simulink model "parallel_controller_mar_10"  (R2017b)
settings: Solver=FixedStepAuto  StartTime=0.0  StopTime=10  FixedStep=0.0001  RelTol=1e-3
InitFcn:
  | ra = 4;
  | jm = 0.0000218;
  | rm = 0.7/100;
  | dsm = 62.892;
  | kt = 0.138;
  | ke = kt;
  | ms = 0.93;
  | hl = 1.5 / 100;
  | Lr = 24.1 / 100;
  | Lcm = hl / 2 + Lr;
  | ml =0.182;
  | mr = 0.085;
  | rl = 20.125 / 1000;
  | Jp =1/3 * mr * Lr^2 + 1/2*ml*rl^2 + ml * Lcm ^ 2;
  | Dp = 0.007;
  | g = 9.82;
StartFcn:
  | ra = 4;
  | jm = 0.0000218;
  | rm = 0.7/100;
  | dsm = 62.892;
  | kt = 0.138;
  | ke = kt;
  | ms = 0.93;
undefined symbols (not defined in the file): direction_sign, distance, Ka, Kd, Ki, Kp, National_Instruments, PCI, saturation_lower, saturation_upper, tau, theta_max
libraries: sldrtlib x4
settings Model: Creator=labadmin  LastModifiedBy=labadmin
settings RTWCC: SystemTargetFile=sldrt.tlc  TemplateMakefile=sldrt.tmf  Description=Simulink Desktop Real-Time  RTWCompilerOptimization=on
settings CodeAppCC: MaxIdLength=95
settings SimulinkDesktopRealTimeCC: TargetPreCompLibLocation=C:\Program Files\MATLAB\R2017b\toolbox\sldrt\lib\win64

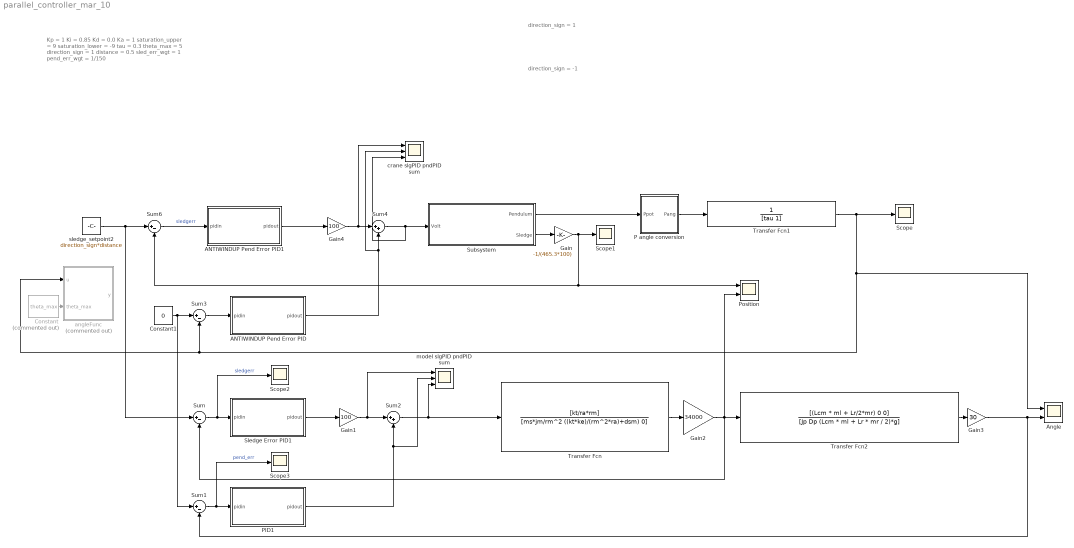
== system parallel_controller_mar_10 ==
  note: Kp = 1
      | Ki = 0.85
      | Kd = 0.0
      | Ka = 1
      | saturation_upper = 9
      | saturation_lower = -9
      | tau = 0.3
      | theta_max = 5
      | direction_sign = 1
      | distance = 0.5
      | sled_err_wgt = 1
      | pend_err_wgt = 1/150
  note: direction_sign = -1
  note: direction_sign = 1
  ANTIWINDUP Pend Error PID : Subsystem
  ANTIWINDUP Pend Error PID1 : Subsystem
  Angle : Scope  NumInputPorts=2
  Constant : Constant  Commented=on  Value=theta_max
  Constant1 : Constant  Value=0
  Gain : Gain  Gain=-1/(465.3*100)
  Gain1 : Gain  Gain=100
  Gain2 : Gain  Gain=34000
  Gain3 : Gain  Gain=30
  Gain4 : Gain  Gain=100
  P angle conversion : Subsystem
  PID1 : Subsystem
  Position : Scope  NumInputPorts=2
  Scope{,1..3} (4 alike) : Scope
  Sledge Error PID1 : Subsystem
  Subsystem : Subsystem
  Sum{,1,3,6} (4 alike) : Sum  Inputs=|+-
  Sum2 : Sum  Inputs=|++
  Sum4 : Sum  Inputs=|++
  Transfer Fcn : TransferFcn  Numerator=[kt/ra*rm]  Denominator=[ms*jm/rm^2 ((kt*ke)/(rm^2*ra)+dsm) 0]
  Transfer Fcn1 : TransferFcn  Denominator=[tau 1]
  Transfer Fcn2 : TransferFcn  Numerator=[(Lcm * ml + Lr/2*mr) 0 0]  Denominator=[Jp Dp (Lcm * ml + Lr * mr / 2)*g]
  "angleFunc " : MATLAB Function  Commented=on  TreatAsAtomicUnit=on
  crane slgPID pndPID sum : Scope  NumInputPorts=3
  model slgPID pndPID sum : Scope  NumInputPorts=3
  sledge_setpoint2 : Constant  Value=direction_sign*distance
  wires:
  Gain/1 -> Sum6/2, Position/1, Scope1/1
  Subsystem/1(Pendulum) -> P angle conversion/1(Ppot)
  Subsystem/2(Sledge) -> Gain/1
  Transfer Fcn/1 -> Gain2/1
  Gain2/1 -> Sum/2, Position/2, Transfer Fcn2/1
  Gain3/1 -> Sum1/2, Angle/2
  sledge_setpoint2/1 -> Sum/1, Sum6/1
  PID1/1(pidout) -> model slgPID pndPID sum/2, Sum2/2
  Sum6/1 -> ANTIWINDUP Pend Error PID1/1(pidin)  "sledgerr"
  P angle conversion/1(Pang) -> Transfer Fcn1/1
  Sum2/1 -> model slgPID pndPID sum/3, Transfer Fcn/1
  Transfer Fcn1/1 -> Scope/1, Angle/1, "angleFunc "/1(u), Sum3/2
  Constant/1 -> "angleFunc "/2(theta_max)
  Constant1/1 -> Sum1/1, Sum3/1
  Transfer Fcn2/1 -> Gain3/1
  Sum3/1 -> ANTIWINDUP Pend Error PID/1(pidin)
  ANTIWINDUP Pend Error PID1/1(pidout) -> Gain4/1
  ANTIWINDUP Pend Error PID/1(pidout) -> crane slgPID pndPID sum/2, Sum4/2
  Sum/1 -> Scope2/1, Sledge Error PID1/1(pidin)  "sledgerr"
  Sledge Error PID1/1(pidout) -> Gain1/1
  Sum1/1 -> Scope3/1, PID1/1(pidin)  "pend_err"
  Gain1/1 -> model slgPID pndPID sum/1, Sum2/1
  Sum4/1 -> crane slgPID pndPID sum/3, Subsystem/1(Volt)
  Gain4/1 -> crane slgPID pndPID sum/1, Sum4/1

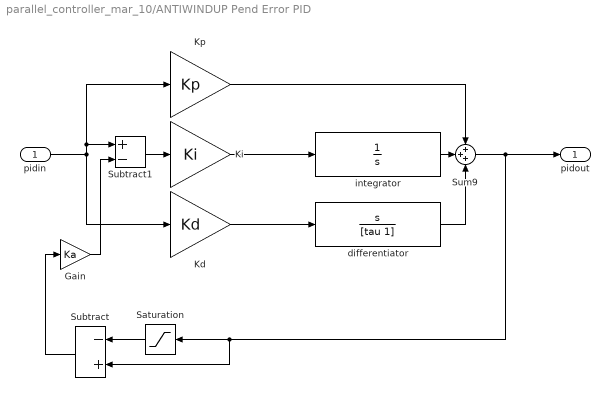
== system parallel_controller_mar_10/ANTIWINDUP Pend Error PID ==
  pidin : Inport
  Gain : Gain  Gain=Ka
  Kd : Gain  Gain=Kd
  Ki : Gain  Gain=Ki
  Kp : Gain  Gain=Kp
  Saturation : Saturate  UpperLimit=saturation_upper  LowerLimit=saturation_lower
  Subtract : Sum  Inputs=-+
  Subtract1 : Sum  Inputs=+-
  Sum9 : Sum  Inputs=+++
  differentiator : TransferFcn  Numerator=[1 0]  Denominator=[tau 1]
  integrator : TransferFcn  Denominator=[1 0]
  pidout : Outport
  wires:
  pidin/1 -> Kp/1, Subtract1/1, Kd/1
  Sum9/1 -> Subtract/2, Saturation/1, pidout/1
  Kd/1 -> differentiator/1
  Ki/1 -> integrator/1
  Kp/1 -> Sum9/1
  integrator/1 -> Sum9/2
  differentiator/1 -> Sum9/3
  Saturation/1 -> Subtract/1
  Subtract/1 -> Gain/1
  Gain/1 -> Subtract1/2
  Subtract1/1 -> Ki/1

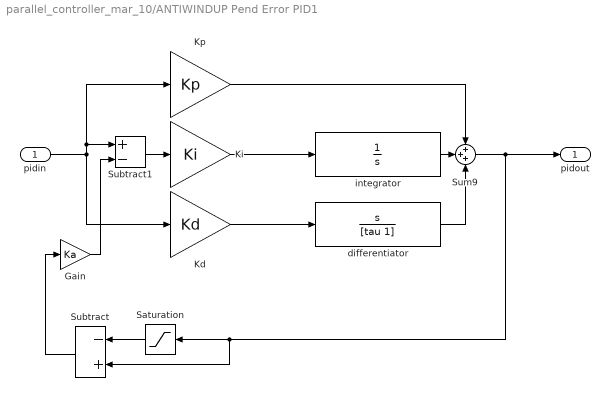
== system parallel_controller_mar_10/ANTIWINDUP Pend Error PID1 ==
  pidin : Inport
  Gain : Gain  Gain=Ka
  Kd : Gain  Gain=Kd
  Ki : Gain  Gain=Ki
  Kp : Gain  Gain=Kp
  Saturation : Saturate  UpperLimit=saturation_upper  LowerLimit=saturation_lower
  Subtract : Sum  Inputs=-+
  Subtract1 : Sum  Inputs=+-
  Sum9 : Sum  Inputs=+++
  differentiator : TransferFcn  Numerator=[1 0]  Denominator=[tau 1]
  integrator : TransferFcn  Denominator=[1 0]
  pidout : Outport
  wires:
  pidin/1 -> Kp/1, Subtract1/1, Kd/1
  Sum9/1 -> Subtract/2, Saturation/1, pidout/1
  Kd/1 -> differentiator/1
  Ki/1 -> integrator/1
  Kp/1 -> Sum9/1
  integrator/1 -> Sum9/2
  differentiator/1 -> Sum9/3
  Saturation/1 -> Subtract/1
  Subtract/1 -> Gain/1
  Gain/1 -> Subtract1/2
  Subtract1/1 -> Ki/1

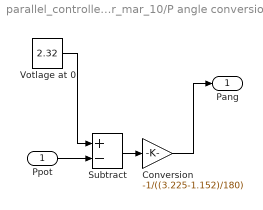
== system parallel_controller_mar_10/P angle conversion ==
  Ppot : Inport
  Conversion : Gain  Gain=-1/((3.225-1.152)/180)
  Subtract : Sum  Inputs=+-
  "Votlage at 0 " : Constant  Value=2.32
  Pang : Outport
  wires:
  Subtract/1 -> Conversion/1
  Ppot/1 -> Subtract/2
  "Votlage at 0 "/1 -> Subtract/1
  Conversion/1 -> Pang/1

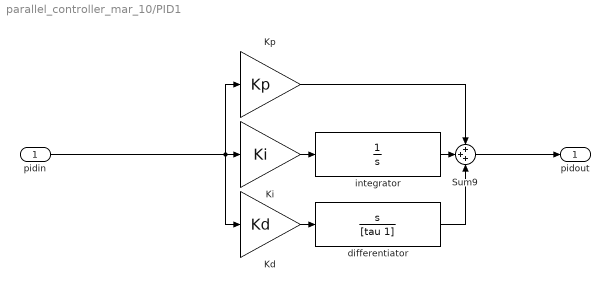
== system parallel_controller_mar_10/PID1 ==
  pidin : Inport
  Kd : Gain  Gain=Kd
  Ki : Gain  Gain=Ki
  Kp : Gain  Gain=Kp
  Sum9 : Sum  Inputs=+++
  differentiator : TransferFcn  Numerator=[1 0]  Denominator=[tau 1]
  integrator : TransferFcn  Denominator=[1 0]
  pidout : Outport
  wires:
  pidin/1 -> Kp/1, Kd/1, Ki/1
  Sum9/1 -> pidout/1
  Kd/1 -> differentiator/1
  Ki/1 -> integrator/1
  Kp/1 -> Sum9/1
  integrator/1 -> Sum9/2
  differentiator/1 -> Sum9/3

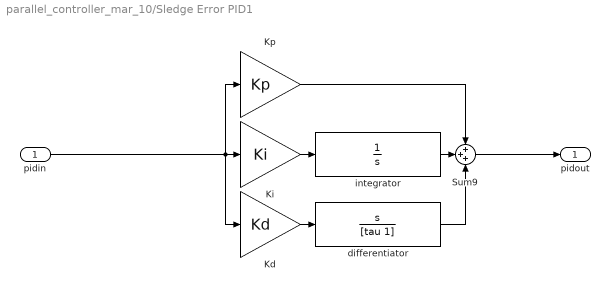
== system parallel_controller_mar_10/Sledge Error PID1 ==
  pidin : Inport
  Kd : Gain  Gain=Kd
  Ki : Gain  Gain=Ki
  Kp : Gain  Gain=Kp
  Sum9 : Sum  Inputs=+++
  differentiator : TransferFcn  Numerator=[1 0]  Denominator=[tau 1]
  integrator : TransferFcn  Denominator=[1 0]
  pidout : Outport
  wires:
  pidin/1 -> Kp/1, Kd/1, Ki/1
  Sum9/1 -> pidout/1
  Kd/1 -> differentiator/1
  Ki/1 -> integrator/1
  Kp/1 -> Sum9/1
  integrator/1 -> Sum9/2
  differentiator/1 -> Sum9/3

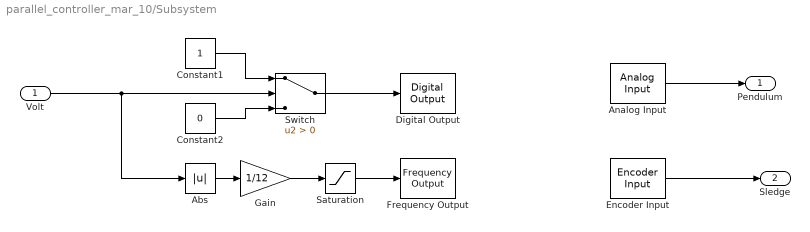
== system parallel_controller_mar_10/Subsystem ==
  Volt : Inport
  Abs : Abs
  Analog Input : sldrtlib/Analog Input  SampleTime=-1  MaxMissedTicks=1000000000  ShowMissedTicks=off  YieldWhenWaiting=off  DrvName=National_Instruments/PCI-6229  DrvAddress=4294967295  DrvOptions=[0 1 8192 2 3]  Channels=1  RangeMode=1  VoltRange=1  DataType=1
      settings: AttributesFormatString=National Instruments\nPCI-6229 [auto]  SourceProductName=Simulink Desktop Real-Time
  Constant1 : Constant
  Constant2 : Constant  Value=0
  Digital Output : sldrtlib/Digital Output  SampleTime=-1  MaxMissedTicks=100000000  ShowMissedTicks=off  YieldWhenWaiting=off  DrvName=National_Instruments/PCI-6229  DrvAddress=4294967295  DrvOptions=[0 1 8192 2 3]  Channels=1  BitMode=1  InitialValue=[]  FinalValue=[]
      settings: AttributesFormatString=National Instruments\nPCI-6229 [auto]  SourceProductName=Simulink Desktop Real-Time  SourceProductBaseCode=WT
  Encoder Input : sldrtlib/Encoder Input  SampleTime=-1  MaxMissedTicks=10000000  ShowMissedTicks=off  YieldWhenWaiting=off  DrvName=National_Instruments/PCI-6229  DrvAddress=4294967295  DrvOptions=[0 1 8192 2 3]  Channels=1  QuadMode=3  IndexPulse=2  InputFilter=Inf  DataType=1
      settings: AttributesFormatString=National Instruments\nPCI-6229 [auto]  SourceProductName=Simulink Desktop Real-Time
  Frequency Output : sldrtlib/Frequency Output  SampleTime=-1  MaxMissedTicks=1000000000  ShowMissedTicks=off  YieldWhenWaiting=off  DrvName=National_Instruments/PCI-6229  DrvAddress=4294967295  DrvOptions=[0 1 8192 2 3]  Channels=2  FrequencySource=1  Frequency=10000  FrequencyFinalValue=[]  DutySource=2  Duty=0  DutyFinalValue=0
      settings: AttributesFormatString=National Instruments\nPCI-6229 [auto]  SourceProductName=Simulink Desktop Real-Time  SourceProductBaseCode=WT
  Gain : Gain  Gain=1/12
  Saturation : Saturate  LowerLimit=0
  Switch : Switch  Criteria=u2 > Threshold
  Pendulum : Outport
  Sledge : Outport  Port=2
  wires:
  Analog Input/1 -> Pendulum/1
  Encoder Input/1 -> Sledge/1
  Saturation/1 -> Frequency Output/1
  Volt/1 -> Abs/1, Switch/2
  Gain/1 -> Saturation/1
  Constant2/1 -> Switch/3
  Abs/1 -> Gain/1
  Constant1/1 -> Switch/1
  Switch/1 -> Digital Output/1

== matlab function parallel_controller_mar_10/angleFunc  ==
  data: u input; y output; theta_max input
function y = angle_setpoint(u, theta_max)
    if (u > theta_max)
        y = u - theta_max;
    elseif u < -theta_max
        y = u + theta_max;
    else
        y = 0;
    end
end
